simulink model "block_sim3"  (R2023b)
settings: Solver=FixedStepAuto  StartTime=0.0  StopTime=10.0  FixedStep=1e-3  RelTol=1e-3
values from neighbouring files (symbols this model uses):
  C1 = 0.0    (= 0)    [simulation3.m]    (also in simulation3_full.m)
  C2 = 0.0    (= 0)    [simulation3.m]    (also in simulation3_full.m)
  Iy = 25000    [simulation3.m]    (also in simulation3_full.m)
  K1 = 0.7*K2    (= 147.374414722)    [simulation3.m]    (also in simulation3_full.m)
  K2 = Ka / 1.7    (= 210.534878174)    [simulation3.m]    (also in simulation3_full.m)
  l1 = 8*12    (= 96)    [simulation3.m]    (also in simulation3_full.m)
  l2 = 8*12    (= 96)    [simulation3.m]    (also in simulation3_full.m)
  ms = Ws / g    (= 9.06594829819)    [simulation3.m]    (also in simulation3_full.m)
  speed = speeds(i)*mph2in_sec    [simulation3_full.m]
settings Model: Creator=adlink  LastModifiedBy=andres
settings OptimizationCC: ReuseModelBlockBuffer=off

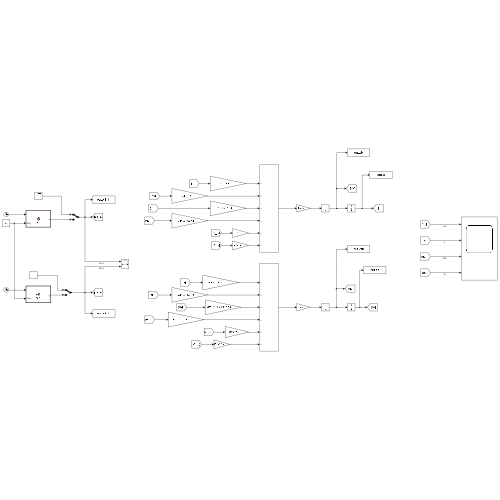
[thumbnail: Simulink's stored preview of the top-level diagram]
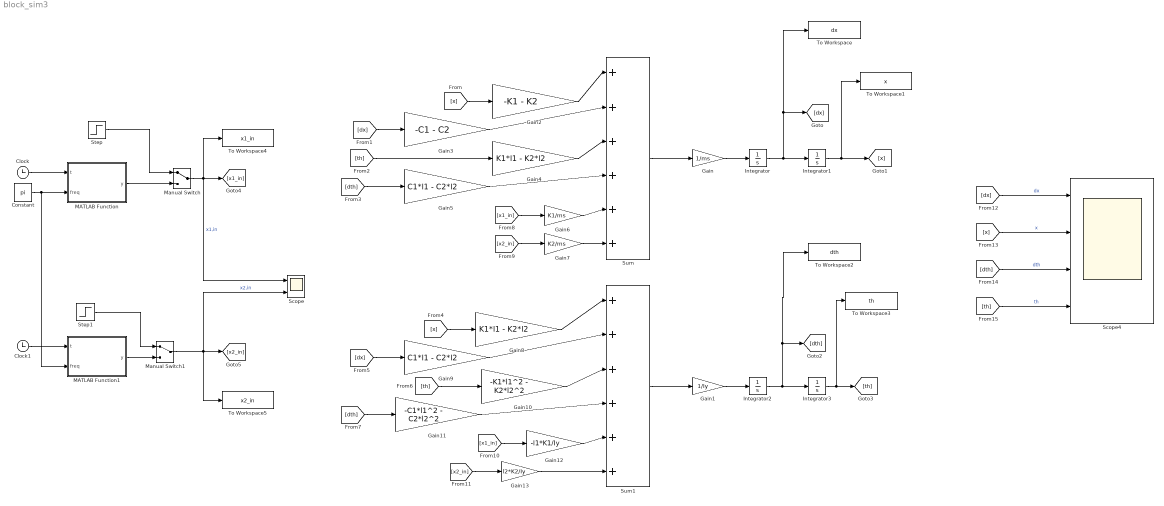
== system block_sim3 ==
  Clock : Clock
  Clock1 : Clock
  Constant : Constant  Value=pi
  Gain : Gain  Gain=1/ms
  Gain1 : Gain  Gain=1/Iy
  Gain10 : Gain  Gain=-K1*l1^2 - K2*l2^2
  Gain11 : Gain  Gain=-C1*l1^2 - C2*l2^2
  Gain12 : Gain  Gain=-l1*K1/Iy
  Gain13 : Gain  Gain=l2*K2/Iy
  Gain2 : Gain  Gain=-K1 - K2
  Gain3 : Gain  Gain=-C1 - C2
  Gain4 : Gain  Gain=K1*l1 - K2*l2
  Gain5 : Gain  Gain=C1*l1 - C2*l2
  Gain6 : Gain  Gain=K1/ms
  Gain7 : Gain  Gain=K2/ms
  Gain8 : Gain  Gain=K1*l1 - K2*l2
  Gain9 : Gain  Gain=C1*l1 - C2*l2
  Integrator{,1..3} (4 alike) : Integrator
  MATLAB Function : MATLAB Function  TreatAsAtomicUnit=on
  MATLAB Function1 : MATLAB Function  TreatAsAtomicUnit=on
  Manual Switch : ManualSwitch
  Manual Switch1 : ManualSwitch
  Scope : Scope  NumInputPorts=2
  Scope4 : Scope  NumInputPorts=4
  Step : Step  SampleTime=0
  Step1 : Step  Time=1 + (l1 + l2)/(speed/0.0568)  SampleTime=0
  Sum : Sum  Inputs=|++++++
  Sum1 : Sum  Inputs=|++++++
  To Workspace : ToWorkspace  VariableName=dx  SaveFormat=Timeseries  SampleTime=0.01
  To Workspace1 : ToWorkspace  VariableName=x  SaveFormat=Timeseries  SampleTime=0.01
  To Workspace2 : ToWorkspace  VariableName=dth  SaveFormat=Timeseries  SampleTime=0.01
  To Workspace3 : ToWorkspace  VariableName=th  SaveFormat=Timeseries  SampleTime=0.01
  To Workspace4 : ToWorkspace  VariableName=x1_in  SaveFormat=Timeseries  SampleTime=0.01
  To Workspace5 : ToWorkspace  VariableName=x2_in  SaveFormat=Timeseries  SampleTime=0.01
  wires:
  Integrator/1 -> [dx], To Workspace/1, Integrator1/1
  Integrator2/1 -> [dth], To Workspace2/1, Integrator3/1
  Gain/1 -> Integrator/1
  Gain1/1 -> Integrator2/1
  Sum/1 -> Gain/1
  Gain2/1 -> Sum/1
  Gain3/1 -> Sum/2
  Gain4/1 -> Sum/3
  Gain5/1 -> Sum/4
  Gain6/1 -> Sum/5
  Gain7/1 -> Sum/6
  Integrator3/1 -> To Workspace3/1, [th]
  Sum1/1 -> Gain1/1
  Gain8/1 -> Sum1/1
  Gain9/1 -> Sum1/2
  Gain10/1 -> Sum1/3
  Gain11/1 -> Sum1/4
  Gain12/1 -> Sum1/5
  Gain13/1 -> Sum1/6
  [x] -> Gain2/1
  [dx] -> Gain3/1
  [th] -> Gain4/1
  [dth] -> Gain5/1
  [x] -> Gain8/1
  [dx] -> Gain9/1
  [th] -> Gain10/1
  [dth] -> Gain11/1
  [x2_in] -> Gain7/1
  [x1_in] -> Gain6/1
  [x2_in] -> Gain13/1
  [x1_in] -> Gain12/1
  Clock/1 -> MATLAB Function/1(t)
  Constant/1 -> MATLAB Function1/2(freq), MATLAB Function/2(freq)
  Manual Switch/1 -> To Workspace4/1, Scope/1, [x1_in]  "x1,in"
  Step/1 -> Manual Switch/1
  MATLAB Function/1(y) -> Manual Switch/2
  Step1/1 -> Manual Switch1/1
  Clock1/1 -> MATLAB Function1/1(t)
  MATLAB Function1/1(y) -> Manual Switch1/2
  Manual Switch1/1 -> To Workspace5/1, Scope/2, [x2_in]  "x2,in"
  Integrator1/1 -> To Workspace1/1, [x]
  [dx] -> Scope4/1  "dx"
  [x] -> Scope4/2  "x"
  [dth] -> Scope4/3  "dth"
  [th] -> Scope4/4  "th"

== matlab function block_sim3/MATLAB Function ==
  data: t input; freq input; y output
function y = fcn(t, freq)
    
    y = sin(freq*t);

    if y > 0
        y = 1;
    else
        y = 0;
    end
end

== matlab function block_sim3/MATLAB Function1 ==
  data: t input; freq input; y output
function y = fcn(t, freq)
    
    y = sin(freq*t+pi);

    if y > 0
        y = 1;
    else
        y = 0;
    end
end
